simulink model "changeEVsoundBackwards"  (R2024b)
settings: Solver=FixedStepDiscrete  StartTime=0.0  StopTime=3  RelTol=1e-3
PreLoadFcn:
  | nsemitones = 3;
libraries: dspsnks4 x1, dspvision x1
settings Model: Creator=ftiong  LastModifiedBy=ftiong
settings SolverCC: AlgebraicLoopSolver=TrustRegion  AutoInsertRateTranBlk=on
settings DataIOCC: LimitDataPoints=on  SaveOutput=off  SignalLogging=off  SaveTime=off
settings OptimizationCC: LifeSpan=inf
settings DebuggingCC: AlgebraicLoopMsg=error  SingleTaskRateTransMsg=error  UnconnectedInputMsg=warning  UnconnectedOutputMsg=warning  UnconnectedLineMsg=warning  AllowSymbolicDim=off  SFUnexpectedBacktrackingDiag=warning  SFNoUnconditionalDefaultTransitionDiag=warning  SFExecutionAtInitializationDiag=none  ArithmeticOperatorsInVariantConditions=warning
settings ModelReferenceCC: EnableRefExpFcnMdlSchedulingChecks=on
settings SFSimCC: SimUseLocalCustomCode=off  CustomCodeUndefinedFunction=UseInterfaceOnly
settings RTWCC: RTWUseLocalCustomCode=off  GPUComputeCapability=3.5
settings CodeAppCC: StateflowObjectComments=on
settings GRTTargetCC: TargetLangStandard=C89/C90 (ANSI)
settings ConfigComp: CovMetricSettings=dw  CovSaveCumulativeToWorkspaceVar=on  CovSaveSingleToWorkspaceVar=on  CovExternalEMLEnable=off  CovSFcnEnable=off

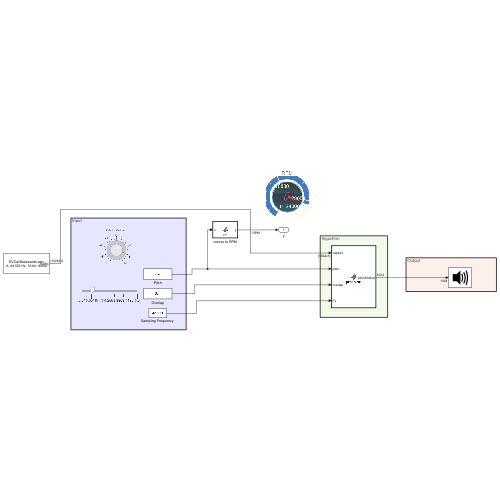
[thumbnail: Simulink's stored preview of the top-level diagram]
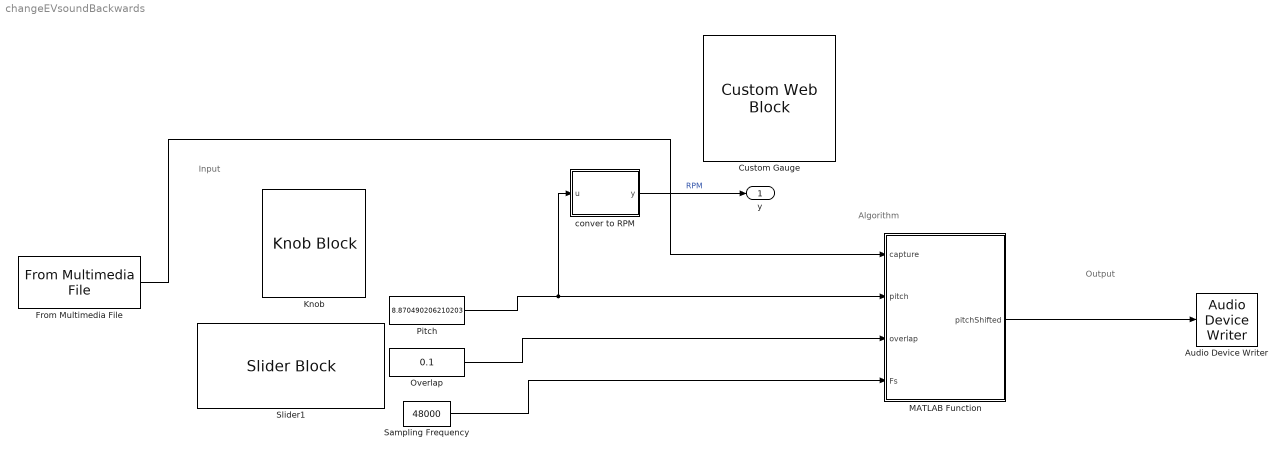
== system changeEVsoundBackwards ==
  note: Algorithm
  note: Output
  note: Input
  Audio Device Writer : dspsnks4/Audio Device Writer  Driver=DirectSound  Device=Default  InheritSampleRate=on  SampleRate=44100  BitDepth=16-bit integer  BufferSize=4096  NumBuffers=10  DefaultOutputChannelMapping=on  OutputChannelMapping=1:2  OutputNumUnderrunSamples=off  DriverIdx=1  DeviceWarnFlag=''
  Custom Gauge : CustomWebBlock  ShowInitialText=on  Configuration="{\"components\":[{\"name\":\"CircularScaleComponent\",\"settings\":{\"bounds\":{\"max\":24000,\"min\":0,\"tickInterval\":\"auto\"},\"direction\":\"cw\",\"flipLimits\":0,\"innerRadius\":0.840457634504587,\"internalTickHeightScaleFactor\":1,\"labelColor\":[250,245,200],\"labelFont\":{\"font\":\"Arial\",\"fontSize\":12},\"labelRadius\":0.5525824738896701,\"labelTransparency\":1,\"minorTickHeightScaleFactor\":0.2,\"needleImage\":{\"size\":[0.18777423402314464,0.11398036452260474],\"src\":\"data:image\\/svg+xml;base64,PD94bWwgdmVyc2lvbj0iMS4wIiBlbmNvZGluZz0idXRmLTgiPz4KPCEtLSBHZW5lcmF0b3I6IEFkb2JlIElsbHVzdHJhdG9yIDE5LjIuMSwgU1ZHIEV4cG9ydCBQbHVnLUluIC4gU1ZHIFZlcnNpb246IDYuMDAgQnVpbGQgMCkgIC0tPgo8c3ZnIHZlcnNpb249IjEuMSIgeG1sbnM9Imh0dHA6Ly93d3cudzMub3JnLzIwMDAvc3ZnIiB4bWxuczp4bGluaz0iaHR0cDovL3d3dy53My5vcmcvMTk5OS94bGluayIgeD0iMHB4IiB5PSIwcHgiCgkgdmlld0JveD0iMCAwIDIwMCA1MCIgc3R5bGU9ImVuYWJsZS1iYWNrZ3JvdW5kOm5ldyAw ...(+9940 chars)\"},\"needleOffset\":[0.09815076084215239,0],\"needleOrientation\":-45,\"needleRotation\":-180,\"needleSize\":{\"height\":0.28495091130651184,\"width\":0.4694355850578616},\"outerRadius\":1.128332795119504,\"position\":[0,0,1,1],\"referencePoint\":\"auto\",\"scaleAngle\":299.999999999988,\"scaleAngleOffset\":119.46147497096791,\"scaleColors\":[],\"scaleColorsSize\":0.2,\"scaleDirection\":\"CW\",\"scalePosition\":[0,0,1,1],\"showLabels\":1,\"showMinorTicks\":1,\"showSpanLine\":1,\"showTicks\":1,\"tickColor\":[250,245,200],\"tickTransparency\":1,\"valueBarColor\":[23,89,176],\"valueBarPosition\":[0,0,1,1],\"valueBarSize\":0.2,\"valueBarTransparency\":1}},{\"name\":\"BackgroundImageComponent\",\"settings\":{\"image\":{\"size\":[0,0],\"src\":\"data:image\\/svg+xml;base64,PD94bWwgdmVyc2lvbj0iMS4wIiBlbmNvZGluZz0iVVRGLTgiIHN0YW5kYWxvbmU9Im5vIj8+CjwhLS0gR2VuZXJhdG9yOiBBZG9iZSBJbGx1c3RyYXRvciAxOS4yLjEsIFNWRyBFeHBvcnQgUGx1Zy1JbiAuIFNWRyBWZXJzaW9uOiA2LjAwIEJ1aWxkIDApICAtLT4KCjxzdmcKICAgeG1sbnM6ZGM9Imh0dHA6Ly9wdXJsLm9yZy9kYy9lbGVtZW50cy8xLjEvIgogICB4bWxuczpjYz0iaHR0cDovL2NyZWF0aXZlY29tbW9ucy5vcmcvbnMjIgogICB4bWxuczpyZGY9Imh0dHA6Ly93d3cudzMub3JnLzE5OTkvMDIvMjItcmRmLXN5bnRh ...(+9660 chars)\",\"srcOrientation\":\"horizontal\"},\"position\":[0,0,1,1],\"scaleMode\":\"0\"}},{\"name\":\"ForegroundImageComponent\",\"settings\":{\"image\":{\"size\":[0,0],\"src\":\"default\",\"srcOrientation\":[]},\"isForeground\":1,\"position\":[0,0,1,1],\"scaleMode\":\"0\"}}],\"settings\":{\"BindingType\":\"signal\",\"backgroundOffset\":0.14,\"backgroundOpacity\":1,\"fixedAspectRatio\":\"on\",\"orientation\":\"horizontal\",\"showBackgroundColor\":0,\"version\":\"R2024b\"},\"type\":\"CircularGauge\"}"
  From Multimedia File : dspvision/From Multimedia File  inputFilename=EVCarBackwards.wav  readRange=[1 Inf]  loop=on  numPlays=inf  outputStreams=Audio only  videoDataType=single  audioDataType=double  inheritSampleTime=on  userDefinedSampleTime=1/30  noAudioOutput=off  isIntensityVideo=off  fourcc=RGB  colorVideoFormat=Separate color signals  outputEOF=off  dataOrg=Column-major  audioFrameSize=1024  computeAudioFrameSize=off  outSamplingMode=Sample based
      settings: LibrarySourceBlock=audiosources/From Multimedia File
  Knob : KnobBlock  ScaleMin=-12  ScaleMax=12
  MATLAB Function : MATLAB Function  TreatAsAtomicUnit=on
  Overlap : Constant  Value=0.1
  "Pitch " : Constant  Value=8.870490206210203
  "Sampling Frequency " : Constant  Value=48000
  Slider1 : SliderBlock  LabelPosition=Hide  ScaleMin=0.01  ScaleMax=0.5
  conver to RPM : MATLAB Function  TreatAsAtomicUnit=on
  y : Outport
  wires:
  From Multimedia File/1 -> MATLAB Function/1(capture)
  "Pitch "/1 -> conver to RPM/1(u), MATLAB Function/2(pitch)
  Overlap/1 -> MATLAB Function/3(overlap)
  "Sampling Frequency "/1 -> MATLAB Function/4(Fs)
  MATLAB Function/1(pitchShifted) -> Audio Device Writer/1
  conver to RPM/1(y) -> y/1  "RPM"

== matlab function changeEVsoundBackwards/conver to RPM ==
  data: u input; y output
function y = fcn(u)

y = (u(1)+12)*1000;

== matlab function changeEVsoundBackwards/MATLAB Function ==
  data: capture input; pitchShifted output; pitch input; overlap input; Fs input
function pitchShifted = pitchShift(capture, pitch, overlap, Fs)
%pitchShift Pitch shift algorithm 
% Copyrights 2018-2019 The MathWorks, Inc.

%#codegen
resetFlag = 0;      % Reset flag set to 0

persistent pitchShifter
if isempty(pitchShifter)
    pitchShifter = audiopluginexample.PitchShifter( ...
        'PitchShift',8,'Overlap',0.3);
    setSampleRate(pitchShifter,Fs);
end

pitchShifted = zeros(size(double(capture)),'like',double(capture));

if nargin > 4 && resetFlag
    reset(pitchShifter);
    return;
end

pitchShifter.PitchShift = pitch;
pitchShifter.Overlap = overlap;

[pitchShifted] = pitchShifter(double(capture));

end
